simulink model "Main_Simulink"  (R2021b)
settings: Solver=VariableStepAuto  StartTime=0.0  StopTime=10.0  RelTol=1e-3
libraries: cstblocks x9, RCTblocks x2, simulink_extras x1
settings Model: Creator=İbrahim  LastModifiedBy=İbrahim

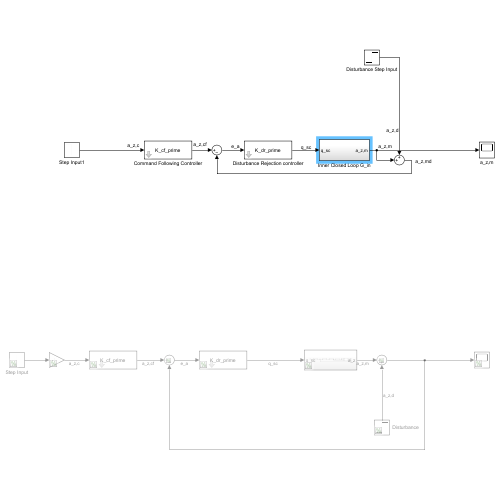
[thumbnail: Simulink's stored preview of the top-level diagram]
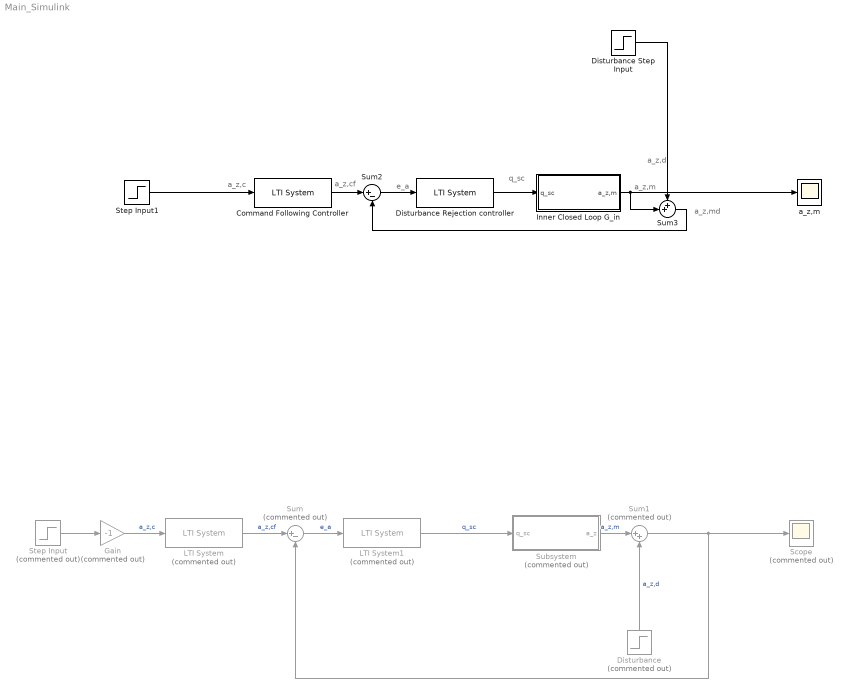
== system Main_Simulink ==
  note: q_sc
  note: e_a
  note: a_z,md
  note: a_z,m
  note: a_z,d
  note: a_z,c
  note: a_z,cf
  Command Following Controller : cstblocks/LTI System  sys=K_cf_prime  IC=[]
  Disturbance : Step  Commented=on  SampleTime=0
  Disturbance Rejection controller : cstblocks/LTI System  sys=K_dr_prime  IC=[]
  Disturbance Step Input : Step  After=0.1  SampleTime=0
  Gain : Gain  Commented=on  Gain=-1
  "Inner Closed Loop G_in " : Subsystem
  LTI System : cstblocks/LTI System  Commented=on  sys=K_cf_prime  IC=[]
  LTI System1 : cstblocks/LTI System  Commented=on  sys=K_dr_prime  IC=[]
  Scope : Scope  Commented=on
  Step Input : Step  Commented=on  SampleTime=0
  Step Input1 : Step  Time=0  After=-1  SampleTime=0
  Subsystem : Subsystem  Commented=on
  Sum : Sum  Commented=on  Inputs=|+-
  Sum1 : Sum  Commented=on  Inputs=|++
  Sum2 : Sum  Inputs=|+-
  Sum3 : Sum  Inputs=++|
  a_z,m : Scope
  wires:
  LTI System1/1 -> Subsystem/1(q_sc)  "q_sc"
  Sum/1 -> LTI System1/1  "e_a"
  LTI System/1 -> Sum/1  "a_z,cf"
  Subsystem/1(a_z) -> Sum1/1  "a_z,m"
  Gain/1 -> LTI System/1  "a_z,c"
  Step Input/1 -> Gain/1
  Disturbance/1 -> Sum1/2  "a_z,d"
  Sum1/1 -> Sum/2, Scope/1
  Step Input1/1 -> Command Following Controller/1
  Disturbance Step Input/1 -> Sum3/1
  Sum2/1 -> Disturbance Rejection controller/1
  Sum3/1 -> Sum2/2
  Disturbance Rejection controller/1 -> "Inner Closed Loop G_in "/1(q_sc)
  Command Following Controller/1 -> Sum2/1
  "Inner Closed Loop G_in "/1(a_z,m) -> Sum3/2, a_z,m/1

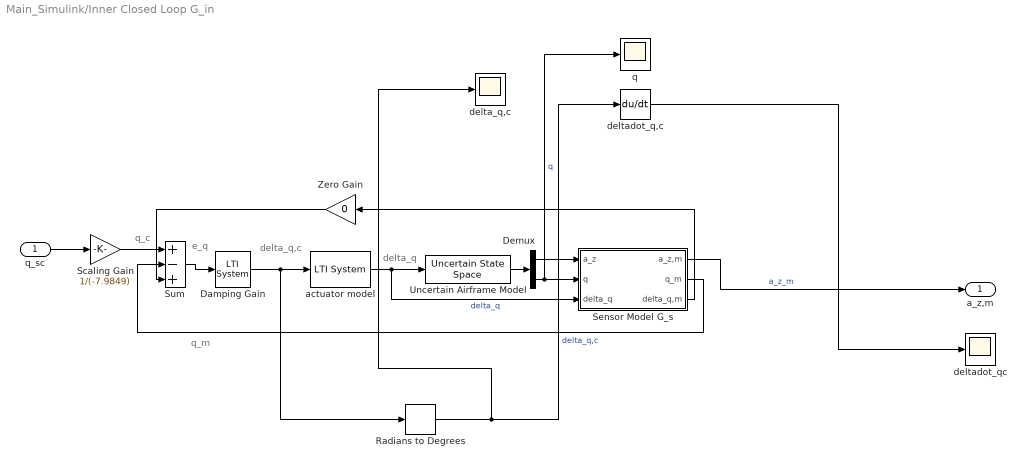
== system Main_Simulink/Inner Closed Loop G_in  ==
  note: q_m
  note: q_c
  note: e_q
  note: delta_q,c
  note: delta_q
  q_sc : Inport
  Damping Gain : cstblocks/LTI System  sys=Kq_sim  IC=[]
  Demux : Demux  Outputs=2
  Radians to Degrees : simulink_extras/Transformations/Radians to Degrees
  Scaling Gain : Gain  Gain=1/(-7.9849)
  Sensor Model G_s : Subsystem
  Sum : Sum  Inputs=+-+
  Uncertain Airframe Model : RCTblocks/Uncertain State Space  Tag=USS  USystem=Gs_af_u  UValue=Gs_af_u.Uncertainty  X0=[]  uX0=[]
      settings: SourceProductBaseCode=RC
  "Zero Gain " : Gain  Gain=0
  actuator model : cstblocks/LTI System  sys=Gs_act  IC=[]
  delta_q,c : Scope
  deltadot_q,c : Derivative
  deltadot_qc : Scope
  q : Scope
  a_z,m : Outport  VectorParamsAs1DForOutWhenUnconnected=off
  wires:
  deltadot_q,c/1 -> deltadot_qc/1
  Radians to Degrees/1 -> delta_q,c/1, deltadot_q,c/1  "delta_q,c"
  Demux/2 -> q/1, Sensor Model G_s/2(q)  "q"
  "Zero Gain "/1 -> Sum/3
  Sensor Model G_s/1(a_z,m) -> a_z,m/1  "a_z_m"
  q_sc/1 -> Scaling Gain/1
  Sensor Model G_s/3(delta_q,m) -> "Zero Gain "/1
  Sensor Model G_s/2(q_m) -> Sum/2
  Demux/1 -> Sensor Model G_s/1(a_z)
  Uncertain Airframe Model/1 -> Demux/1
  Sum/1 -> Damping Gain/1
  actuator model/1 -> Uncertain Airframe Model/1, Sensor Model G_s/3(delta_q)  "delta_q"
  Damping Gain/1 -> Radians to Degrees/1, actuator model/1
  Scaling Gain/1 -> Sum/1

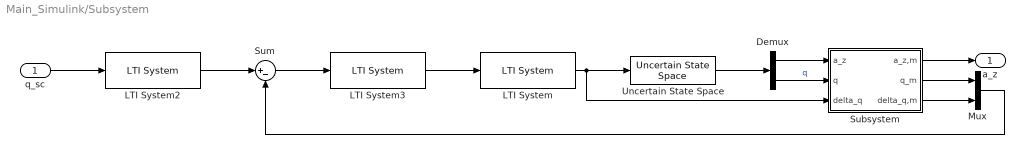
== system Main_Simulink/Subsystem ==
  q_sc : Inport
  Demux : Demux  Outputs=2
  LTI System : cstblocks/LTI System  sys=Gs_act  IC=[]
  LTI System2 : cstblocks/LTI System  sys=Ksc_sim  IC=[]
  LTI System3 : cstblocks/LTI System  sys=Kq_sim  IC=[]
  Mux : Mux  Inputs=2
  Subsystem : Subsystem
  Sum : Sum  Inputs=|+-
  Uncertain State Space : RCTblocks/Uncertain State Space  Tag=USS  USystem=Gs_af_u  UValue=Gs_af_u.Uncertainty  X0=[]  uX0=[]
      settings: SourceProductBaseCode=RC
  a_z : Outport
  wires:
  q_sc/1 -> LTI System2/1
  LTI System2/1 -> Sum/1
  LTI System3/1 -> LTI System/1
  LTI System/1 -> Uncertain State Space/1, Subsystem/3(delta_q)
  Uncertain State Space/1 -> Demux/1
  Demux/2 -> Subsystem/2(q)  "q"
  Demux/1 -> Subsystem/1(a_z)
  Subsystem/2(q_m) -> Mux/1
  Subsystem/3(delta_q,m) -> Mux/2
  Mux/1 -> Sum/2
  Subsystem/1(a_z,m) -> a_z/1
  Sum/1 -> LTI System3/1

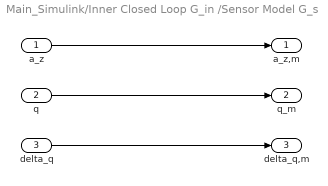
== system Main_Simulink/Inner Closed Loop G_in /Sensor Model G_s ==
  a_z : Inport
  q : Inport  Port=2
  delta_q : Inport  Port=3
  a_z,m : Outport  VectorParamsAs1DForOutWhenUnconnected=off
  q_m : Outport  Port=2  VectorParamsAs1DForOutWhenUnconnected=off
  delta_q,m : Outport  Port=3  VectorParamsAs1DForOutWhenUnconnected=off
  wires:
  delta_q/1 -> delta_q,m/1
  q/1 -> q_m/1
  a_z/1 -> a_z,m/1

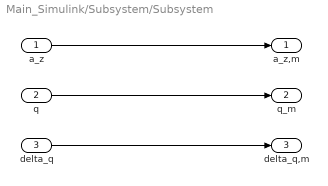
== system Main_Simulink/Subsystem/Subsystem ==
  a_z : Inport
  q : Inport  Port=2
  delta_q : Inport  Port=3
  a_z,m : Outport
  q_m : Outport  Port=2
  delta_q,m : Outport  Port=3
  wires:
  a_z/1 -> a_z,m/1
  q/1 -> q_m/1
  delta_q/1 -> delta_q,m/1
